simulink model "target_transmit"  (R2018a)
settings: Solver=FixedStepDiscrete  StartTime=0  StopTime=inf  RelTol=1e-3  EnableMultiTasking=on
InitFcn:
  | load data/bestsimulink_data
  | load data/bestsimulink320x240_data
  | load busObjects
StopFcn:
  | clear bestsimulink320x240_data
  | clear bestsimulink_data
  | clear dataBusObject
model workspace (MAT data in the model file):
  dt = 0.1
undefined symbols (not defined in the file or in its folder): gray, IsPositionTracked, IsSkeletonTracked, JointDepthIndices, JointImageIndices, JointTrackingState, JointWorldCoordinates, none, PositionDepthIndices, PositionImageIndices, PositionWorldCoordinates, Rec, SDTV, SegmentationData, SkeletonTrackingID, videoinput
libraries: visiontextngfix x24, embdlinuxlib x13, visionstatistics x7, visionconversions x5, visiontransforms x3, visionsinks x2, visionanalysis x1, dspvision x1, imaqlib x1, sldrtlib x1
(part 1 of 2)
settings Model: PauseTimes=118.9  ExtModeTrigDuration=100  Creator=sbiagion  LastModifiedBy=Farwa
settings DataIOCC: LimitDataPoints=on  SaveFormat=StructureWithTime
settings OptimizationCC: LifeSpan=1
settings DebuggingCC: UnderspecifiedInitializationDetection=Classic  MergeDetectMultiDrivingBlocksExec=none  SFUnexpectedBacktrackingDiag=warning  SFNoUnconditionalDefaultTransitionDiag=warning  SFExecutionAtInitializationDiag=none
settings HardwareCC: ProdBitPerPointer=32  ProdBitPerSizeT=32  ProdBitPerPtrDiffT=32  ProdLargestAtomicInteger=Long  ProdLargestAtomicFloat=Double  ProdIntDivRoundTo=Undefined  ProdWordSize=32  ProdHWDeviceType=ARM Compatible->ARM Cortex
settings ModelReferenceCC: PropagateSignalLabelsOutOfModel=off
settings SFSimCC: MATLABDynamicMemAlloc=off
settings RTWCC: SystemTargetFile=realtime.tlc  GenerateMakefile=off  TemplateMakefile=realtime.tmf  Description=Run on Target Hardware  RTWVerbose=off
settings CodeAppCC: StateflowObjectComments=on
settings STFCustomTargetCC: TargetLibSuffix=.a  GenerateSampleERTMain=on  ERTCustomFileBanners=on  SupportNonInlinedSFcns=off  RemoveResetFunc=on  SupportVariableSizeSignals=on  MATLABClassNameForMDSCustomization=Simulink.SoftwareTarget.ERTCustomization  GRTInterface=off  SystemTargetFile=realtime.tlc
settings ERTTargetCC: MultiwordLength=2048  GenerateSampleERTMain=on  ParMdlRefBuildCompliant=off  CompOptLevelCompliant=off  ConcurrentExecutionCompliant=off  CombineOutputUpdateFcns=off  SupportContinuousTime=on  SupportVariableSizeSignals=on  ModelStepFunctionPrototypeControlCompliant=off  CPPClassGenCompliant=off  UseToolchainInfoCompliant=off  ExtMode=on  ExtModeMexArgs='10.10.10.101' 0 17725  ERTSrcFileBannerTemplate=realtime_code_template.cgt  ERTHdrFileBannerTemplate=realtime_code_template.cgt  ERTDataSrcFileTemplate=realtime_code_template.cgt  ERTDataHdrFileTemplate=realtime_code_template.cgt  ERTCustomFileTemplate=realtime_file_process.tlc  ConvertIfToSwitch=off  SuppressUnreachableDefaultCases=off
settings ConfigComp: CovMetricSettings=dw  CovHtmlReporting=on  CovSaveCumulativeToWorkspaceVar=on  CovSaveSingleToWorkspaceVar=on  CovExternalEMLEnable=off

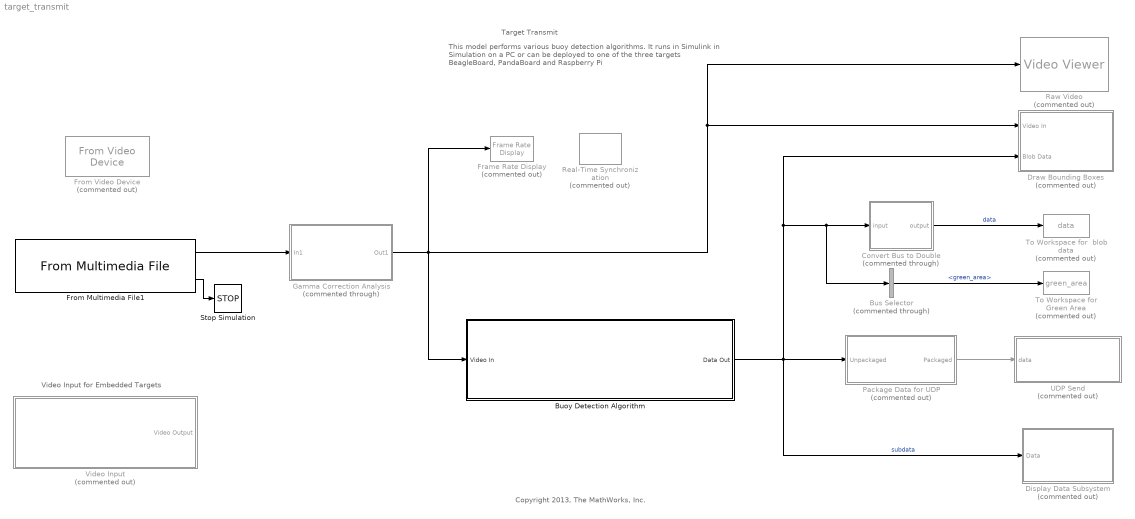
== system target_transmit ==
  note: This model performs various buoy detection algorithms.
      | It runs in Simulink in Simulation on a PC or can be deployed
      |  to one of the three targets BeagleBoard, PandaBoard and Raspberry Pi
  note: Target Transmit
  note: Copyright 2013, The MathWorks, Inc.
  note: Video Input for Embedded Targets
  Buoy Detection Algorithm : Subsystem  Variant=on  OverrideUsingVariant=testControl
  Bus Selector : BusSelector  Commented=through  OutputSignals=green_area
  Convert Bus to Double : Subsystem  Commented=through
  Display Data Subsystem : Subsystem  Commented=on
  Draw Bounding Boxes : Subsystem  Commented=on
  Frame Rate Display : visionsinks/Frame Rate Display  Commented=on  UpdateRate=10
      settings: SourceProductName=Computer Vision System Toolbox  SourceProductBaseCode=VP
  From Multimedia File1 : dspvision/From Multimedia File  inputFilename=E:\Actual_Computer_Stuff\Documents\RoboSoccer\soccer-vision\media\videos\2.mp4  loop=on  numPlays=1  outputStreams=Video only  videoDataType=single  audioDataType=int16  inheritSampleTime=on  userDefinedSampleTime=0.1  noAudioOutput=off  isIntensityVideo=off  fourcc=Intensity  colorVideoFormat=One multidimensional signal  outputEOF=on  dataOrg=Column-major  audioFrameSize=1024  computeAudioFrameSize=off  outSamplingMode=Sample based
      settings: SourceProductBaseCode=VP
  From Video Device : imaqlib/From Video Device  Commented=on  DeviceMenu=(none)  Device=winvideo 1 (Microsoft LifeCam Cinema)  ObjConstructor=videoinput('winvideo', 1)  VideoFormatMenu=(none)  VideoFormat=MJPG_640x480  VideoSource=input1  ROIPosition=[0 0 480 640]  EnableHWTrigger=off  TriggerConfiguration=none/none  SampleTime=0.1  OutputPortsMode=One multidimensional signal  DataType=single  CanDoHWTrigger=no  ReturnedColorSpace=rgb  BlockHandle=2792.0001  ROIWidth=640  ROIHeight=480  ROIColumn=0  ROIRow=0  EngXMLPath=C:\Program Files\MATLAB\R2018a\toolbox\imaq\imaq\private  DevXMLPath=C:\Program Files\MATLAB\R2015a\toolbox\imaq\imaqadaptors\win64  EngLibPath=C:\Program Files\MATLAB\R2018a\toolbox\imaq\imaqblks\imaqmex\win64  ColorSpace=rgb  BayerSensorAlignment=grbg  AllMetadata=IsPositionTracked;IsSkeletonTracked;JointDepthIndices;JointImageIndices;JointTrackingState;JointWorldCoordinates;PositionDepthIndices;PositionImageIndices;PositionWorldCoordinates;SegmentationData;SkeletonTrackingID
      settings: SourceProductName=Image Acquisition Toolbox
  Gamma Correction Analysis : Subsystem  Commented=through
  Package Data for UDP : Subsystem  Commented=on
  "Raw Video " : VideoViewer  Commented=on  colormapValue=gray(256)  FigPos=[1206 549 664 431]
  Real-Time Synchronization : sldrtlib/Real-Time Synchronization  Commented=on  SampleTime=0.1  MaxMissedTicks=1e9  ShowMissedTicks=off  YieldWhenWaiting=off
  Stop Simulation : Stop
  To Workspace for  blob data : ToWorkspace  Commented=on  VariableName=data  SaveFormat=Timeseries  SampleTime=-1
  To Workspace for Green Area : ToWorkspace  Commented=on  VariableName=green_area  SaveFormat=Structure With Time  SampleTime=-1
  UDP Send : Subsystem  Commented=on  Variant=on  OverrideUsingVariant=variantBeagle
  Video Input : Subsystem  Commented=on  Variant=on  OverrideUsingVariant=variantBeagle640x480
  wires:
  From Multimedia File1/2 -> Stop Simulation/1
  Buoy Detection Algorithm/1(Data Out) -> Draw Bounding Boxes/2(Blob Data), Bus Selector/1, Convert Bus to Double/1(input), Display Data Subsystem/1(Data), Package Data for UDP/1(Unpackaged)  "subdata"
  Convert Bus to Double/1(output) -> To Workspace for  blob data/1  "data"
  From Multimedia File1/1 -> Gamma Correction Analysis/1(In1)
  Gamma Correction Analysis/1(Out1) -> Frame Rate Display/1, "Raw Video "/1, Draw Bounding Boxes/1(Video In), Buoy Detection Algorithm/1(Video In)
  Package Data for UDP/1(Packaged) -> UDP Send/1(data)
  Bus Selector/1 -> To Workspace for Green Area/1  "<green_area>"

== system target_transmit/Buoy Detection Algorithm ==
  note: Lower and Upper Bound Thresholding for HSV
      | Multiple Threshold Sets
      | Simulink
      | - Thresholding
      | - Closing
      | - Blob Analysis
  note: Subtraction Based Thresholding in RGB
      | Simulink
      | - Thresholding
      | - Blob Analysis
      | - Limited to 4 Blobs
  note: Lower and Upper Bound Thresholding for RGB
      | Multiple Threshold Sets
      | Matlab Function Block
      | - Thresholding
      | - Closing
      | - Blob Analysis
  note: Lower and Upper Bound Based Thresholding for RGB
      | Multiple Threshold Sets
      | Matlab Function Block
      | - Thresholding
      | - Blob Analysis
  note: Lower and Upper Bound Based Thresholding for RGB
      | Multiple Threshold Sets
      | Simulink
      | - Thresholding
      | - Blob Analysis
  note: Lower and Upper Bound Based Thresholding for RGB
      | Single Threshold Set
      | Simulink
      | - Thresholding
      | - Blob Analysis
  note: Lower and Upper Bound Thresholding for RGB
      | Multiple Threshold Sets
      | Simulink
      | - Thresholding
      | - Closing
      | - Blob Analysis
  note: Subtraction Based Thresholding in RGB
      | Simulink
      | - Thresholding
      | - Blob Analysis
      | - Limited to 50 Blobs
  Video In : Inport
  variant1: Subtraction Based Thresholding 4 Blobs : Subsystem  VariantControl=testControl
  Data Out : Outport

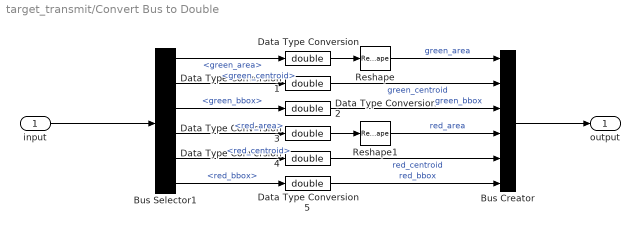
== system target_transmit/Convert Bus to Double ==
  input : Inport
  Bus Creator : BusCreator  Inputs=6
  Bus Selector1 : BusSelector  OutputSignals=green_area,green_centroid,green_bbox,red_area,red_centroid,red_bbox
  Data Type Conversion{,1..5} (6 alike) : DataTypeConversion  OutDataTypeStr=double
  Reshape : Reshape
  Reshape1 : Reshape
  output : Outport
  wires:
  Bus Creator/1 -> output/1
  input/1 -> Bus Selector1/1
  Bus Selector1/4 -> Data Type Conversion3/1  "<red_area>"
  Bus Selector1/6 -> Data Type Conversion5/1  "<red_bbox>"
  Bus Selector1/5 -> Data Type Conversion4/1  "<red_centroid>"
  Bus Selector1/2 -> Data Type Conversion1/1  "<green_centroid>"
  Bus Selector1/3 -> Data Type Conversion2/1  "<green_bbox>"
  Bus Selector1/1 -> Data Type Conversion/1  "<green_area>"
  Data Type Conversion/1 -> Reshape/1
  Data Type Conversion1/1 -> Bus Creator/2  "green_centroid"
  Data Type Conversion2/1 -> Bus Creator/3  "green_bbox"
  Data Type Conversion3/1 -> Reshape1/1
  Data Type Conversion4/1 -> Bus Creator/5  "red_centroid"
  Data Type Conversion5/1 -> Bus Creator/6  "red_bbox"
  Reshape/1 -> Bus Creator/1  "green_area"
  Reshape1/1 -> Bus Creator/4  "red_area"

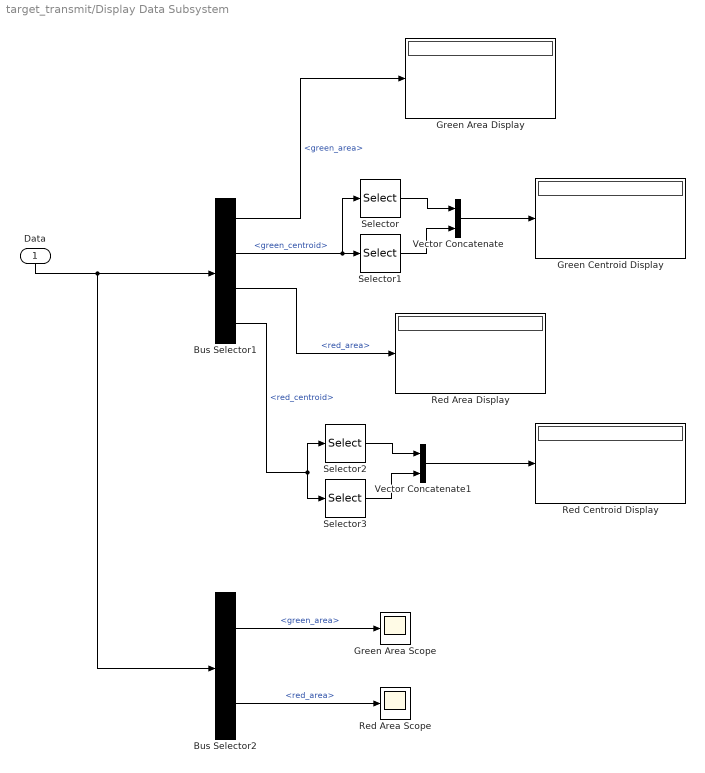
== system target_transmit/Display Data Subsystem ==
  Data : Inport
  Bus Selector1 : BusSelector  OutputSignals=green_area,green_centroid,red_area,red_centroid
  Bus Selector2 : BusSelector  OutputSignals=green_area,red_area
  Green Area Display : Display
  Green Area Scope : Scope
  Green Centroid Display : Display
  Red Area Display : Display
  Red Area Scope : Scope
  Red Centroid Display : Display
  Selector : Selector  NumberOfDimensions=2  InputPortWidth=3  IndexOptions=Select all,Index vector (dialog)  Indices=[1 3],2  OutputSizes=1,1
  Selector1 : Selector  NumberOfDimensions=2  InputPortWidth=3  IndexOptions=Select all,Index vector (dialog)  Indices=[1 3],1  OutputSizes=1,1
  Selector2 : Selector  NumberOfDimensions=2  InputPortWidth=3  IndexOptions=Select all,Index vector (dialog)  Indices=[1 3],2  OutputSizes=1,1
  Selector3 : Selector  NumberOfDimensions=2  InputPortWidth=3  IndexOptions=Select all,Index vector (dialog)  Indices=[1 3],1  OutputSizes=1,1
  Vector Concatenate : Concatenate  Mode=Multidimensional array  ConcatenateDimension=2
  Vector Concatenate1 : Concatenate  Mode=Multidimensional array  ConcatenateDimension=2
  wires:
  Data/1 -> Bus Selector2/1, Bus Selector1/1
  Bus Selector1/1 -> Green Area Display/1  "<green_area>"
  Bus Selector1/2 -> Selector1/1, Selector/1  "<green_centroid>"
  Bus Selector1/3 -> Red Area Display/1  "<red_area>"
  Bus Selector2/1 -> Green Area Scope/1  "<green_area>"
  Bus Selector2/2 -> Red Area Scope/1  "<red_area>"
  Selector/1 -> Vector Concatenate/1
  Selector1/1 -> Vector Concatenate/2
  Vector Concatenate/1 -> Green Centroid Display/1
  Bus Selector1/4 -> Selector3/1, Selector2/1  "<red_centroid>"
  Selector2/1 -> Vector Concatenate1/1
  Selector3/1 -> Vector Concatenate1/2
  Vector Concatenate1/1 -> Red Centroid Display/1

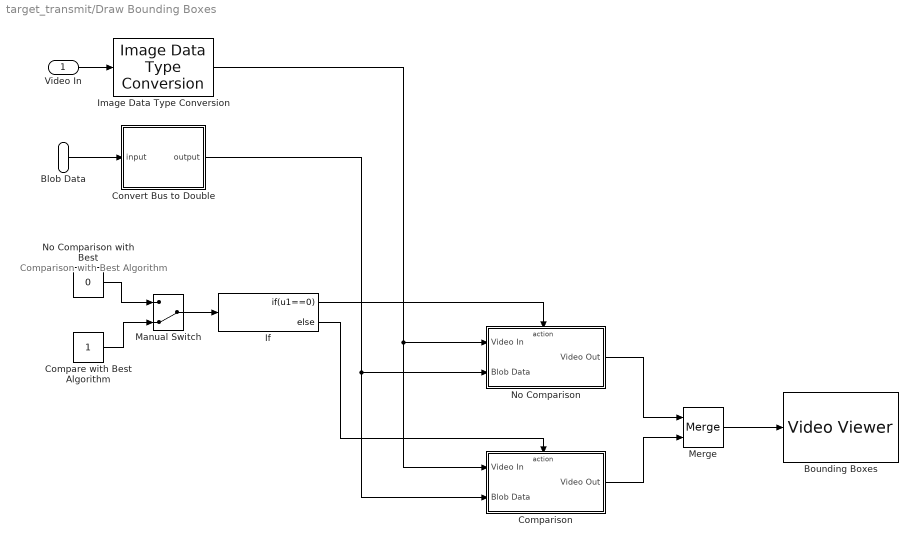
== system target_transmit/Draw Bounding Boxes ==
  note: Comparison with Best Algorithm
  Video In : Inport
  Blob Data : Inport  Port=2
  Bounding Boxes : VideoViewer  colormapValue=gray(256)  FigPos=[1 678 1280 582.666666666667]
  Compare with Best Algorithm : Constant
  Comparison : Subsystem  TreatAsAtomicUnit=on
  Convert Bus to Double : Subsystem
  If : If  IfExpression=u1==0
  Image Data Type Conversion : visionconversions/Image Data Type Conversion  outDT=double  isSigned=on  wordLen=16  numFracBits=0
      settings: SourceProductName=Computer Vision System Toolbox  SourceProductBaseCode=VP
  Manual Switch : ManualSwitch  CurrentSetting=0
  Merge : Merge
  No Comparison : Subsystem  TreatAsAtomicUnit=on
  No Comparison with Best : Constant  Value=0
  wires:
  Video In/1 -> Image Data Type Conversion/1
  Blob Data/1 -> Convert Bus to Double/1(input)
  Convert Bus to Double/1(output) -> No Comparison/2(Blob Data), Comparison/2(Blob Data)
  No Comparison with Best/1 -> Manual Switch/1
  Compare with Best Algorithm/1 -> Manual Switch/2
  Manual Switch/1 -> If/1
  If/1 -> No Comparison/Action
  Image Data Type Conversion/1 -> Comparison/1(Video In), No Comparison/1(Video In)
  If/2 -> Comparison/Action
  No Comparison/1(Video Out) -> Merge/1
  Comparison/1(Video Out) -> Merge/2
  Merge/1 -> Bounding Boxes/1

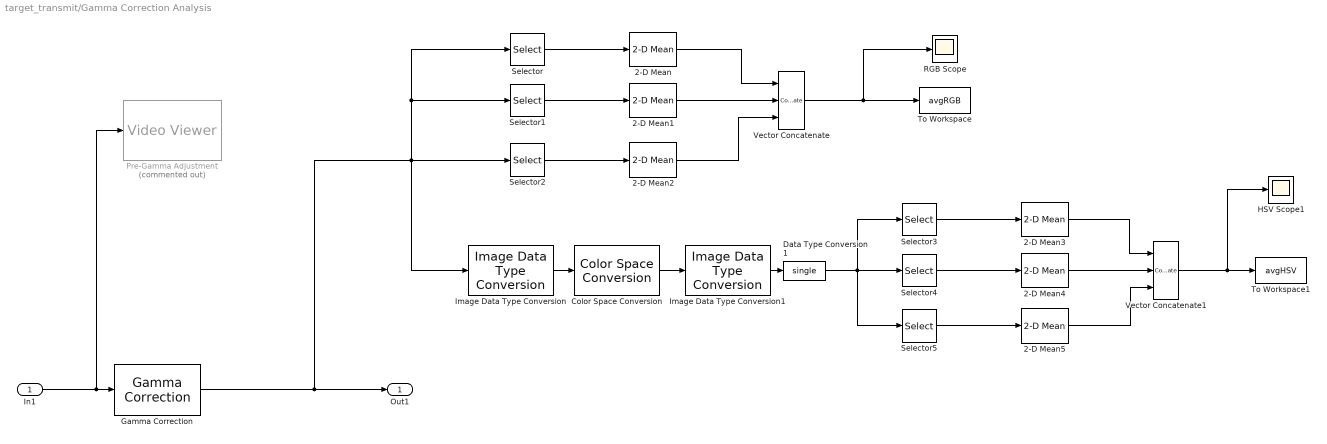
== system target_transmit/Gamma Correction Analysis ==
  In1 : Inport
  2-D Mean{,1..5} (6 alike) : visionstatistics/2-D Mean  run=off  reset_popup=None  directionMode=Entire input  dimension=1  treatSBRowAsCol=on  roiEnable=off  roiType=Rectangles  roiPortion=Entire ROI  roiOutput=Individual statistics for each ROI  roiFlag=off  outputDataTypeStr=Inherit: Same as accumulator  outputLastDataTypeStr=Inherit: Same as accumulator  outputMin=[]  outputMax=[]  accumMode=Binary point scaling  accumWordLength=32  accumFracLength=0  accumDataTypeStr=fixdt([],32,0)  accumLastDataTypeStr=fixdt([],32,0)  roundingMode=Floor  overflowMode=off
      settings: SourceProductName=Computer Vision System Toolbox  SourceProductBaseCode=VP
  Color Space Conversion : visionconversions/Color Space  Conversion  conversion=Obsolete  conversionActive=R'G'B' to HSV  wp_str=D65  rec=Rec. 601 (SDTV)  sys=1125/60/2:1  imagePorts=One multidimensional signal
      settings: SourceProductName=Computer Vision System Toolbox
  Data Type Conversion1 : DataTypeConversion  OutDataTypeStr=single  SaturateOnIntegerOverflow=on  RndMeth=Zero
  Gamma Correction : visionconversions/Gamma Correction  operation=Gamma  gamma=1.5  linearSegment=on  breakPoint=0.018
      settings: SourceProductName=Computer Vision System Toolbox  SourceProductBaseCode=VP
  HSV Scope1 : Scope
  Image Data Type Conversion : visionconversions/Image Data Type Conversion  outDT=single  isSigned=on  wordLen=16  numFracBits=0
      settings: SourceProductName=Computer Vision System Toolbox  SourceProductBaseCode=VP
  Image Data Type Conversion1 : visionconversions/Image Data Type Conversion  outDT=uint8  isSigned=on  wordLen=16  numFracBits=0
      settings: SourceProductName=Computer Vision System Toolbox  SourceProductBaseCode=VP
  Pre-Gamma Adjustment : visionsinks/Video Viewer  Commented=on  inputType=Obsolete7b  imagePorts=One multidimensional signal  useColorMap=off  colormapValue=gray(256)  specRange=off  minInputVal=0  maxInputVal=255  FigPos=[119 991 1008 708]  AxisZoom=on  trueSizedOnce=off  OpenAtMdlStart=on  DefaultConfigurationName=vipscopes.VideoViewerScopeCfg
      settings: SourceProductName=Computer Vision System Toolbox  SourceProductBaseCode=VP
  RGB Scope : Scope
  Selector : Selector  NumberOfDimensions=3  InputPortWidth=3  IndexOptions=Select all,Select all,Index vector (dialog)  Indices=[1 3],1,1  OutputSizes=1,1,1
  Selector1 : Selector  NumberOfDimensions=3  InputPortWidth=3  IndexOptions=Select all,Select all,Index vector (dialog)  Indices=[1 3],1,2  OutputSizes=1,1,1
  Selector2 : Selector  NumberOfDimensions=3  InputPortWidth=3  IndexOptions=Select all,Select all,Index vector (dialog)  Indices=[1 3],1,3  OutputSizes=1,1,1
  Selector3 : Selector  NumberOfDimensions=3  InputPortWidth=3  IndexOptions=Select all,Select all,Index vector (dialog)  Indices=[1 3],1,1  OutputSizes=1,1,1
  Selector4 : Selector  NumberOfDimensions=3  InputPortWidth=3  IndexOptions=Select all,Select all,Index vector (dialog)  Indices=[1 3],1,2  OutputSizes=1,1,1
  Selector5 : Selector  NumberOfDimensions=3  InputPortWidth=3  IndexOptions=Select all,Select all,Index vector (dialog)  Indices=[1 3],1,3  OutputSizes=1,1,1
  To Workspace : ToWorkspace  VariableName=avgRGB  SaveFormat=Timeseries  SampleTime=-1
  To Workspace1 : ToWorkspace  VariableName=avgHSV  SaveFormat=Timeseries  SampleTime=-1
  Vector Concatenate : Concatenate  NumInputs=3
  Vector Concatenate1 : Concatenate  NumInputs=3
  Out1 : Outport
  wires:
  In1/1 -> Pre-Gamma Adjustment/1, Gamma Correction/1
  Gamma Correction/1 -> Selector2/1, Selector1/1, Selector/1, Image Data Type Conversion/1, Out1/1
  Selector1/1 -> 2-D Mean1/1
  Selector2/1 -> 2-D Mean2/1
  Selector/1 -> 2-D Mean/1
  2-D Mean/1 -> Vector Concatenate/1
  2-D Mean1/1 -> Vector Concatenate/2
  2-D Mean2/1 -> Vector Concatenate/3
  Vector Concatenate/1 -> To Workspace/1, RGB Scope/1
  Color Space Conversion/1 -> Image Data Type Conversion1/1
  Image Data Type Conversion/1 -> Color Space Conversion/1
  Data Type Conversion1/1 -> Selector5/1, Selector3/1, Selector4/1
  2-D Mean3/1 -> Vector Concatenate1/1
  2-D Mean4/1 -> Vector Concatenate1/2
  2-D Mean5/1 -> Vector Concatenate1/3
  Vector Concatenate1/1 -> HSV Scope1/1, To Workspace1/1
  Selector3/1 -> 2-D Mean3/1
  Selector4/1 -> 2-D Mean4/1
  Selector5/1 -> 2-D Mean5/1
  Image Data Type Conversion1/1 -> Data Type Conversion1/1

== system target_transmit/Package Data for UDP ==
  Unpackaged : Inport
  Bus Selector : BusSelector  OutputSignals=green_area,green_centroid,red_area,red_centroid
  Mux : Mux
  Reshape1 : Reshape
  Reshape2 : Reshape
  Packaged : Outport
  wires:
  Mux/1 -> Packaged/1
  Bus Selector/1 -> Mux/1  "<green_area>"
  Bus Selector/2 -> Reshape2/1  "<green_centroid>"
  Bus Selector/3 -> Mux/3  "<red_area>"
  Bus Selector/4 -> Reshape1/1  "<red_centroid>"
  Reshape2/1 -> Mux/2
  Reshape1/1 -> Mux/4
  Unpackaged/1 -> Bus Selector/1

== system target_transmit/UDP Send ==
  data : Inport
  UDP Send BeagleBoard : Subsystem  VariantControl=variantBeagle
  UDP Send PandaBoard : Subsystem  VariantControl=variantPanda
  UDP Send RaspberryPi : Subsystem  VariantControl=variantRPi

== system target_transmit/Video Input ==
  variant1: BeagleBoard 640x480 : Subsystem  VariantControl=variantBeagle640x480
  variant2: BeagleBoard 320x240 : Subsystem  VariantControl=variantBeagle320x240
  variant3: PandaBoard 640x480 : Subsystem  VariantControl=variantPanda640x480
  variant4: PandaBoard 320x240 : Subsystem  VariantControl=variantPanda320x240
  variant5: RasbPi 320x240 : Subsystem  VariantControl=variantRasbPi320x240
  Video Output : Outport

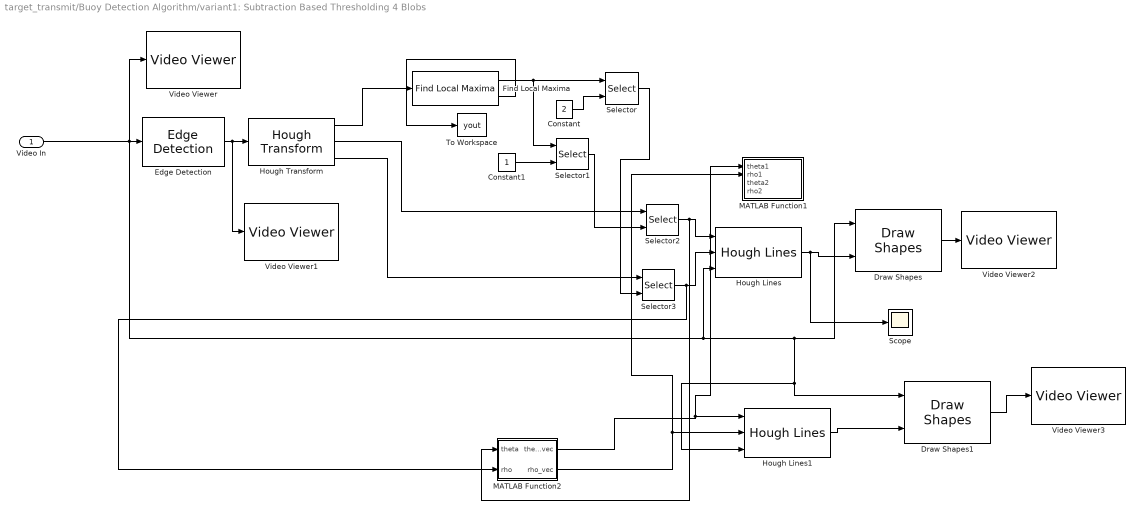
== system target_transmit/Buoy Detection Algorithm/variant1: Subtraction Based Thresholding 4 Blobs ==
  Video In : Inport
  Constant : Constant  Value=2
  Constant1 : Constant
  Draw Shapes : visiontextngfix/Draw Shapes  shape=Lines  fill=off  lineWidth=8  fillClrSource=Specify via dialog  display=White  intensity=200  color=[0 128 0]  opacity=0.6  viewport=Entire image  antialiasing=off  inType=Obsolete  imagePorts=One multidimensional signal  prodOutputMode=Binary point scaling  prodOutputWordLength=32  prodOutputFracLength=14  memoryMode=Specify word length  memoryWordLength=16  memoryFracLength=14  roundingMode=Floor  overflowMode=off
      settings: SourceProductName=Computer Vision System Toolbox
  Draw Shapes1 : visiontextngfix/Draw Shapes  shape=Lines  fill=off  lineWidth=8  fillClrSource=Specify via dialog  display=Black  intensity=200  color=[0 128 0]  opacity=0.6  viewport=Entire image  antialiasing=off  inType=Obsolete  imagePorts=One multidimensional signal  prodOutputMode=Binary point scaling  prodOutputWordLength=32  prodOutputFracLength=14  memoryMode=Specify word length  memoryWordLength=16  memoryFracLength=14  roundingMode=Floor  overflowMode=off
      settings: SourceProductName=Computer Vision System Toolbox
  Edge Detection : visionanalysis/Edge Detection  method=Sobel  outputType=Binary image  userDefinedThreshold=off  thresholdSource=Input port  threshold=20  thresholdTuning=12  edgeThinning=off  threshold_canny=[0.25 0.60]  autoPercent=70  sigma=1  roundingMode=Floor  overflowMode=off  prodOutputMode=Binary point scaling  prodOutputWordLength=32  prodOutputFracLength=8  prodOutputSlope=2^-8  accumSlope=2^-8  outputSlope=2^-4
      settings: SourceProductName=Computer Vision System Toolbox  SourceProductBaseCode=VP
  Find Local Maxima : visionstatistics/Find Local Maxima  num_peaks=8  nhood_size=[5 7]  src_thresh=Obsolete9b  src_thresh_inuse=Specify via dialog  threshold=10  inputIsHough=on  dt_peak=uint32  isOutVarDim=off  dt_count=uint32
      settings: SourceProductName=Computer Vision System Toolbox  SourceProductBaseCode=VP
  Hough Lines : visiontransforms/Hough Lines  sineCompMethod=Trigonometric function  thetaRes=pi/180  firstCoeffMode=Specify word length  firstCoeffWordLength=16  firstCoeffFracLength=15  prodOutputMode=Binary point scaling  prodOutputWordLength=32  prodOutputFracLength=16  roundingMode=Nearest  overflowMode=on
      settings: SourceProductName=Computer Vision System Toolbox  SourceProductBaseCode=VP
  Hough Lines1 : visiontransforms/Hough Lines  sineCompMethod=Trigonometric function  thetaRes=pi/180  firstCoeffMode=Specify word length  firstCoeffWordLength=16  firstCoeffFracLength=15  prodOutputMode=Binary point scaling  prodOutputWordLength=32  prodOutputFracLength=16  roundingMode=Nearest  overflowMode=on
      settings: SourceProductName=Computer Vision System Toolbox  SourceProductBaseCode=VP
  Hough Transform : visiontransforms/Hough Transform  theta_res=pi/360  rho_res=1  out_theta_rho=on  outdtmode=double  firstCoeffMode=Binary point scaling  firstCoeffWordLength=16  firstCoeffFracLength=14  secondCoeffMode=Binary point scaling  secondCoeffWordLength=32  secondCoeffFracLength=16  outputMode=Binary point scaling  outputWordLength=16  outputFracLength=0  accumMode=Binary point scaling  accumWordLength=32  accumFracLength=20  prodOutputMode=Binary point scaling  prodOutputWordLength=32  prodOutputFracLength=20  memoryMode=Binary point scaling  memoryWordLength=32  memoryFracLength=16  roundingMode=Nearest  overflowMode=on
      settings: SourceProductName=Computer Vision System Toolbox  SourceProductBaseCode=VP
  MATLAB Function1 : MATLAB Function  TreatAsAtomicUnit=on
  MATLAB Function2 : MATLAB Function  TreatAsAtomicUnit=on
  Scope : Scope
  Selector : Selector  NumberOfDimensions=2  InputPortWidth=2  IndexOptions=Select all,Index vector (port)  Indices=1,1  OutputSizes=1,1
  Selector1 : Selector  NumberOfDimensions=2  InputPortWidth=2  IndexOptions=Select all,Index vector (port)  Indices=0,1  OutputSizes=1,1
  Selector2 : Selector  NumberOfDimensions=2  InputPortWidth=3  IndexOptions=Select all,Index vector (port)  Indices=[1 3],1  OutputSizes=1,1
  Selector3 : Selector  NumberOfDimensions=2  InputPortWidth=3  IndexOptions=Select all,Index vector (port)  Indices=[1 3],1  OutputSizes=1,1
  To Workspace : ToWorkspace  VariableName=yout  SampleTime=-1
      settings: Save2DSignal=2-D array (concatenate along first dimension)
  Video Viewer : VideoViewer  colormapValue=gray(256)  FigPos=[1 678 1280 582.666666666667]
  Video Viewer1 : VideoViewer  colormapValue=gray(256)  FigPos=[1 678 1280 582.666666666667]
  Video Viewer2 : VideoViewer  colormapValue=gray(256)  FigPos=[503.666666666667 715.333333333333 638.666666666667 574.666666666667]
  Video Viewer3 : VideoViewer  colormapValue=gray(256)  FigPos=[-11.6666666666667 725.333333333333 1280 582.666666666667]
  wires:
  Constant1/1 -> Selector1/2
  Video In/1 -> Edge Detection/1, Hough Lines/3, Draw Shapes1/1, Hough Lines1/3, Draw Shapes/1, Video Viewer/1
  Hough Lines/1 -> Scope/1, Draw Shapes/2
  Selector/1 -> Selector3/2
  Selector1/1 -> Selector2/2
  Draw Shapes/1 -> Video Viewer2/1
  Find Local Maxima/1 -> Selector1/1, Selector/1
  Hough Transform/2 -> Selector2/1
  Constant/1 -> Selector/2
  Edge Detection/1 -> Hough Transform/1, Video Viewer1/1
  Hough Transform/1 -> Find Local Maxima/1
  Find Local Maxima/2 -> To Workspace/1
  Selector3/1 -> MATLAB Function2/2(rho), Hough Lines/2
  Selector2/1 -> MATLAB Function2/1(theta), Hough Lines/1
  Hough Transform/3 -> Selector3/1
  Draw Shapes1/1 -> Video Viewer3/1
  Hough Lines1/1 -> Draw Shapes1/2
  MATLAB Function2/1(theta_vec) -> MATLAB Function1/1(theta1), Hough Lines1/1
  MATLAB Function2/2(rho_vec) -> MATLAB Function1/2(rho1), Hough Lines1/2

== system target_transmit/Draw Bounding Boxes/Comparison ==
  Video In : Inport
  Blob Data : Inport  Port=2
  Action Port : ActionPort  ActionType=else
  Insert Algorithm Blobs : Subsystem
  Insert Area Text : Subsystem  Commented=through
  Insert Best Algorithm Blobs : Subsystem
  Insert Closest Text : Subsystem
  Insert Speed Gate or Buoy Text : Subsystem  Commented=through
  Reflection Removal : Subsystem  Commented=through
  Video Out : Outport
  wires:
  Blob Data/1 -> Reflection Removal/1(Blob Data In)
  Video In/1 -> Insert Best Algorithm Blobs/1(Video In)
  Insert Best Algorithm Blobs/1(Video Out) -> Insert Closest Text/1(Video In)
  Reflection Removal/1(Blob Data Out) -> Insert Area Text/2(Blob Data)
  Insert Closest Text/1(Video Out) -> Insert Area Text/1(Video In)
  Insert Area Text/1(Video Out) -> Insert Speed Gate or Buoy Text/1(Video In)
  Insert Speed Gate or Buoy Text/1(Video Out) -> Insert Algorithm Blobs/1(Video In)
  Insert Algorithm Blobs/1(Video Out) -> Video Out/1
  Insert Speed Gate or Buoy Text/2(Data output) -> Insert Algorithm Blobs/2(Blob Data)
  Insert Area Text/2(Blob Data Out) -> Insert Speed Gate or Buoy Text/2(Blob Data)
  Insert Best Algorithm Blobs/2(Best Data Out) -> Insert Closest Text/2(Blob Data)

== system target_transmit/Draw Bounding Boxes/Convert Bus to Double ==
  input : Inport
  Bus Creator : BusCreator  Inputs=6
  Bus Selector1 : BusSelector  OutputSignals=green_area,green_centroid,green_bbox,red_area,red_centroid,red_bbox
  Data Type Conversion{,1..5} (6 alike) : DataTypeConversion  OutDataTypeStr=double
  output : Outport
  wires:
  Bus Creator/1 -> output/1
  input/1 -> Bus Selector1/1
  Bus Selector1/4 -> Data Type Conversion3/1  "<red_area>"
  Bus Selector1/6 -> Data Type Conversion5/1  "<red_bbox>"
  Bus Selector1/5 -> Data Type Conversion4/1  "<red_centroid>"
  Bus Selector1/2 -> Data Type Conversion1/1  "<green_centroid>"
  Bus Selector1/3 -> Data Type Conversion2/1  "<green_bbox>"
  Bus Selector1/1 -> Data Type Conversion/1  "<green_area>"
  Data Type Conversion1/1 -> Bus Creator/2  "green_centroid"
  Data Type Conversion2/1 -> Bus Creator/3  "green_bbox"
  Data Type Conversion4/1 -> Bus Creator/5  "red_centroid"
  Data Type Conversion5/1 -> Bus Creator/6  "red_bbox"
  Data Type Conversion/1 -> Bus Creator/1  "green_area"
  Data Type Conversion3/1 -> Bus Creator/4  "red_area"

== system target_transmit/Draw Bounding Boxes/No Comparison ==
  Video In : Inport
  Blob Data : Inport  Port=2
  Action Port : ActionPort  ActionType=then
  Insert Area Text : Subsystem  Commented=through
  Insert Buoy Blobs1 : Subsystem
  Insert Closest Text : Subsystem
  Insert Speed Gate or Buoy Text : Subsystem  Commented=through
  Reflection Removal : Subsystem  Commented=through
  Video Out : Outport
  wires:
  Insert Area Text/1(Video Out) -> Insert Speed Gate or Buoy Text/1(Video In)
  Insert Closest Text/1(Video Out) -> Insert Area Text/1(Video In)
  Insert Speed Gate or Buoy Text/1(Video Out) -> Video Out/1
  Reflection Removal/1(Blob Data Out) -> Insert Buoy Blobs1/2(Blob Data), Insert Area Text/2(Blob Data), Insert Closest Text/2(Blob Data)
  Insert Buoy Blobs1/1(Video Out) -> Insert Closest Text/1(Video In)
  Video In/1 -> Insert Buoy Blobs1/1(Video In)
  Blob Data/1 -> Reflection Removal/1(Blob Data In)
  Insert Area Text/2(Blob Data Out) -> Insert Speed Gate or Buoy Text/2(Blob Data)

== system target_transmit/UDP Send/UDP Send BeagleBoard ==
  data : Inport
  UDP Send : embdlinuxlib/UDP Send  remoteURL='10.10.10.100'  remotePort=25001  localURL='255.255.255.255'  localPortSource=Automatically determine  localPort=-1  sampletime=-1  blockPlatform=BeagleBoard  separateLengthPort=0
      settings: SourceProductName=Simulink Support Package for Raspberry Pi Hardware  SourceProductBaseCode=RASPPI
  wires:
  data/1 -> UDP Send/1

== system target_transmit/UDP Send/UDP Send PandaBoard ==
  data : Inport
  UDP Send1 : embdlinuxlib/UDP Send  remoteURL='10.10.10.100'  remotePort=25001  localURL='255.255.255.255'  localPortSource=Automatically determine  localPort=-1  sampletime=-1  blockPlatform=PandaBoard  separateLengthPort=0
      settings: SourceProductName=Simulink Support Package for Raspberry Pi Hardware  SourceProductBaseCode=RASPPI
  wires:
  data/1 -> UDP Send1/1

== system target_transmit/UDP Send/UDP Send RaspberryPi ==
  data : Inport
  UDP Send2 : embdlinuxlib/UDP Send  remoteURL='172.28.65.74'  remotePort=25000  localURL='255.255.255.255'  localPortSource=Automatically determine  localPort=-1  sampletime=-1  blockPlatform=Raspberry Pi  separateLengthPort=0
      settings: SourceProductName=Simulink Support Package for Raspberry Pi Hardware  SourceProductBaseCode=RASPPI
  wires:
  data/1 -> UDP Send2/1

== system target_transmit/Video Input/variant1: BeagleBoard 640x480 ==
  SDL Video Display : embdlinuxlib/SDL Video Display  Commented=on  pixelFormat=RGB  pixelOrder=Planar  rowMajor=on  blockPlatform=BeagleBoard
      settings: SourceProductName=Simulink Support Package for Raspberry Pi Hardware  SourceProductBaseCode=RASPPI
  V4L2 Video Capture : embdlinuxlib/V4L2 Video Capture  m_devName='/dev/video0'  roi=[0, 0, 640, 480]  imSizeSelection=640x480  imSize=[640, 480]  pixelFormat=RGB  pixelOrder=Planar  sampleTime=0.1  simOutput=Colorbars  blockPlatform=BeagleBoard
      settings: SourceProductName=Simulink Support Package for Raspberry Pi Hardware  SourceProductBaseCode=RASPPI
  Vector Concatenate : Concatenate  NumInputs=3  Mode=Multidimensional array  ConcatenateDimension=3
  Video Output : Outport
  wires:
  Vector Concatenate/1 -> Video Output/1
  V4L2 Video Capture/1 -> SDL Video Display/1, Vector Concatenate/1
  V4L2 Video Capture/2 -> SDL Video Display/2, Vector Concatenate/2
  V4L2 Video Capture/3 -> SDL Video Display/3, Vector Concatenate/3

== system target_transmit/Video Input/variant2: BeagleBoard 320x240 ==
  SDL Video Display : embdlinuxlib/SDL Video Display  pixelFormat=RGB  pixelOrder=Planar  rowMajor=on  blockPlatform=BeagleBoard
      settings: SourceProductName=Simulink Support Package for Raspberry Pi Hardware  SourceProductBaseCode=RASPPI
  V4L2 Video Capture : embdlinuxlib/V4L2 Video Capture  m_devName='/dev/video0'  roi=[0, 0, 640, 480]  imSizeSelection=320x240  imSize=[640, 480]  pixelFormat=RGB  pixelOrder=Planar  sampleTime=0.1  simOutput=Colorbars  blockPlatform=BeagleBoard
      settings: SourceProductName=Simulink Support Package for Raspberry Pi Hardware  SourceProductBaseCode=RASPPI
  Vector Concatenate : Concatenate  NumInputs=3  Mode=Multidimensional array  ConcatenateDimension=3
  Video Output : Outport
  wires:
  V4L2 Video Capture/3 -> Vector Concatenate/3, SDL Video Display/3
  V4L2 Video Capture/2 -> Vector Concatenate/2, SDL Video Display/2
  V4L2 Video Capture/1 -> Vector Concatenate/1, SDL Video Display/1
  Vector Concatenate/1 -> Video Output/1

== system target_transmit/Video Input/variant3: PandaBoard 640x480 ==
  SDL Video Display : embdlinuxlib/SDL Video Display  pixelFormat=RGB  pixelOrder=Planar  rowMajor=on  blockPlatform=PandaBoard
      settings: SourceProductName=Simulink Support Package for Raspberry Pi Hardware  SourceProductBaseCode=RASPPI
  V4L2 Video Capture1 : embdlinuxlib/V4L2 Video Capture  m_devName='/dev/video3'  roi=[0, 0, 640, 480]  imSizeSelection=640x480  imSize=[640, 480]  pixelFormat=RGB  pixelOrder=Planar  sampleTime=0.1  simOutput=Colorbars  blockPlatform=PandaBoard
      settings: SourceProductName=Simulink Support Package for Raspberry Pi Hardware  SourceProductBaseCode=RASPPI
  Vector Concatenate1 : Concatenate  NumInputs=3  Mode=Multidimensional array  ConcatenateDimension=3
  Video Output : Outport
  wires:
  Vector Concatenate1/1 -> Video Output/1
  V4L2 Video Capture1/3 -> SDL Video Display/3, Vector Concatenate1/3
  V4L2 Video Capture1/1 -> SDL Video Display/1, Vector Concatenate1/1
  V4L2 Video Capture1/2 -> SDL Video Display/2, Vector Concatenate1/2

== system target_transmit/Video Input/variant4: PandaBoard 320x240 ==
  SDL Video Display : embdlinuxlib/SDL Video Display  pixelFormat=RGB  pixelOrder=Planar  rowMajor=on  blockPlatform=PandaBoard
      settings: SourceProductName=Simulink Support Package for Raspberry Pi Hardware  SourceProductBaseCode=RASPPI
  V4L2 Video Capture1 : embdlinuxlib/V4L2 Video Capture  m_devName='/dev/video3'  roi=[0, 0, 640, 480]  imSizeSelection=320x240  imSize=[640, 480]  pixelFormat=RGB  pixelOrder=Planar  sampleTime=0.5  simOutput=Colorbars  blockPlatform=PandaBoard
      settings: SourceProductName=Simulink Support Package for Raspberry Pi Hardware  SourceProductBaseCode=RASPPI
  Vector Concatenate1 : Concatenate  NumInputs=3  Mode=Multidimensional array  ConcatenateDimension=3
  Video Output : Outport
  wires:
  V4L2 Video Capture1/2 -> Vector Concatenate1/2, SDL Video Display/2
  V4L2 Video Capture1/1 -> Vector Concatenate1/1, SDL Video Display/1
  V4L2 Video Capture1/3 -> Vector Concatenate1/3, SDL Video Display/3
  Vector Concatenate1/1 -> Video Output/1

== system target_transmit/Video Input/variant5: RasbPi 320x240 ==
  SDL Video Display1 : embdlinuxlib/SDL Video Display  pixelFormat=RGB  pixelOrder=Planar  rowMajor=on  blockPlatform=Raspberry Pi
      settings: SourceProductName=Simulink Support Package for Raspberry Pi Hardware  SourceProductBaseCode=RASPPI
  V4L2 Video Capture2 : embdlinuxlib/V4L2 Video Capture  m_devName='/dev/video0'  roi=[0, 0, 640, 480]  imSizeSelection=320x240  imSize=[640, 480]  pixelFormat=RGB  pixelOrder=Planar  sampleTime=0.1  simOutput=Colorbars  blockPlatform=Raspberry Pi
      settings: SourceProductName=Simulink Support Package for Raspberry Pi Hardware  SourceProductBaseCode=RASPPI
  Vector Concatenate2 : Concatenate  NumInputs=3  Mode=Multidimensional array  ConcatenateDimension=3
  Video Output : Outport
  wires:
  V4L2 Video Capture2/1 -> Vector Concatenate2/1, SDL Video Display1/1
  V4L2 Video Capture2/2 -> Vector Concatenate2/2, SDL Video Display1/2
  V4L2 Video Capture2/3 -> Vector Concatenate2/3, SDL Video Display1/3
  Vector Concatenate2/1 -> Video Output/1

== system target_transmit/Draw Bounding Boxes/Comparison/Insert Algorithm Blobs ==
  Video In : Inport
  Blob Data : Inport  Port=2
  Bus Selector : BusSelector  OutputSignals=green_bbox,red_bbox
  Draw Shapes Green : visiontextngfix/Draw Shapes  shape=Rectangles  fill=off  lineWidth=1  fillClrSource=Specify via dialog  display=Black  intensity=200  color=[0 255 0]  opacity=0.6  viewport=Entire image  antialiasing=off  inType=Obsolete  imagePorts=One multidimensional signal  prodOutputMode=Binary point scaling  prodOutputWordLength=32  prodOutputFracLength=14  memoryMode=Specify word length  memoryWordLength=16  memoryFracLength=14  roundingMode=Floor  overflowMode=off
      settings: SourceProductName=Computer Vision System Toolbox
  Draw Shapes Red : visiontextngfix/Draw Shapes  shape=Rectangles  fill=off  lineWidth=1  fillClrSource=Specify via dialog  display=Black  intensity=200  color=[255 0 0]  opacity=0.6  viewport=Entire image  antialiasing=off  inType=Obsolete  imagePorts=One multidimensional signal  prodOutputMode=Binary point scaling  prodOutputWordLength=32  prodOutputFracLength=14  memoryMode=Specify word length  memoryWordLength=16  memoryFracLength=14  roundingMode=Floor  overflowMode=off
      settings: SourceProductName=Computer Vision System Toolbox
  Video Out : Outport
  wires:
  Bus Selector/2 -> Draw Shapes Red/2  "<red_bbox>"
  Bus Selector/1 -> Draw Shapes Green/2  "<green_bbox>"
  Draw Shapes Red/1 -> Video Out/1
  Draw Shapes Green/1 -> Draw Shapes Red/1
  Video In/1 -> Draw Shapes Green/1
  Blob Data/1 -> Bus Selector/1

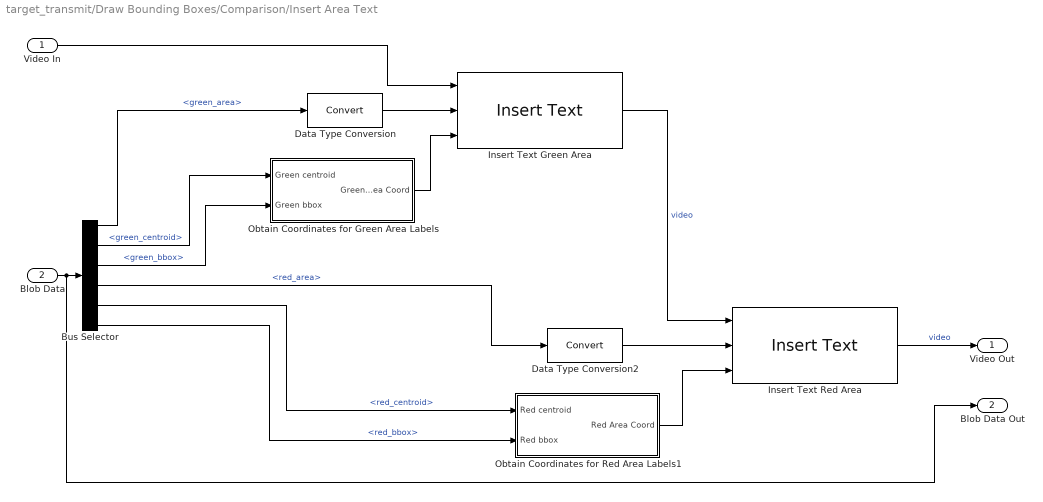
== system target_transmit/Draw Bounding Boxes/Comparison/Insert Area Text ==
  Video In : Inport
  Blob Data : Inport  Port=2
  Bus Selector : BusSelector  OutputSignals=green_area,green_centroid,green_bbox,red_area,red_centroid,red_bbox
  Data Type Conversion : DataTypeConversion
  Data Type Conversion2 : DataTypeConversion
  Insert Text Green Area : visiontextngfix/Insert Text  inputType=Obsolete  theText='Area: %d'  fontFace=LucidaSansRegular  dummyVar1=0  blockFontSize=12  antiAliased=on  getTextLocFrom=Input port  textLoc=[1 1]  getTextColorFrom=Specify via dialog  textColor=[0 255 0]  getTextIntensityFrom=Specify via dialog  textIntensity=0  getTextOpacityFrom=Specify via dialog  textOpacity=1.0  dummyVar2=0  dummyVar3=0  dummyVar4=0  imagePorts=One multidimensional signal  isInputTransposed=off
      settings: SourceProductName=Computer Vision System Toolbox  SourceProductBaseCode=VP
  Insert Text Red Area : visiontextngfix/Insert Text  inputType=Obsolete  theText='Area: %d'  fontFace=LucidaSansRegular  dummyVar1=0  blockFontSize=12  antiAliased=on  getTextLocFrom=Input port  textLoc=[1 1]  getTextColorFrom=Specify via dialog  textColor=[255 0 0]  getTextIntensityFrom=Specify via dialog  textIntensity=0  getTextOpacityFrom=Specify via dialog  textOpacity=1.0  dummyVar2=0  dummyVar3=0  dummyVar4=0  imagePorts=One multidimensional signal  isInputTransposed=off
      settings: SourceProductName=Computer Vision System Toolbox  SourceProductBaseCode=VP
  Obtain Coordinates for Green Area Labels : Subsystem
  Obtain Coordinates for Red Area Labels1 : Subsystem
  Video Out : Outport
  Blob Data Out : Outport  Port=2
  wires:
  Bus Selector/6 -> Obtain Coordinates for Red Area Labels1/2(Red bbox)  "<red_bbox>"
  Bus Selector/5 -> Obtain Coordinates for Red Area Labels1/1(Red centroid)  "<red_centroid>"
  Bus Selector/3 -> Obtain Coordinates for Green Area Labels/2(Green bbox)  "<green_bbox>"
  Bus Selector/2 -> Obtain Coordinates for Green Area Labels/1(Green centroid)  "<green_centroid>"
  Blob Data/1 -> Blob Data Out/1, Bus Selector/1
  Obtain Coordinates for Green Area Labels/1(Green Area Coord) -> Insert Text Green Area/3
  Data Type Conversion2/1 -> Insert Text Red Area/2
  Insert Text Green Area/1 -> Insert Text Red Area/1  "video"
  Obtain Coordinates for Red Area Labels1/1(Red Area Coord) -> Insert Text Red Area/3
  Data Type Conversion/1 -> Insert Text Green Area/2
  Bus Selector/1 -> Data Type Conversion/1  "<green_area>"
  Bus Selector/4 -> Data Type Conversion2/1  "<red_area>"
  Video In/1 -> Insert Text Green Area/1
  Insert Text Red Area/1 -> Video Out/1  "video"

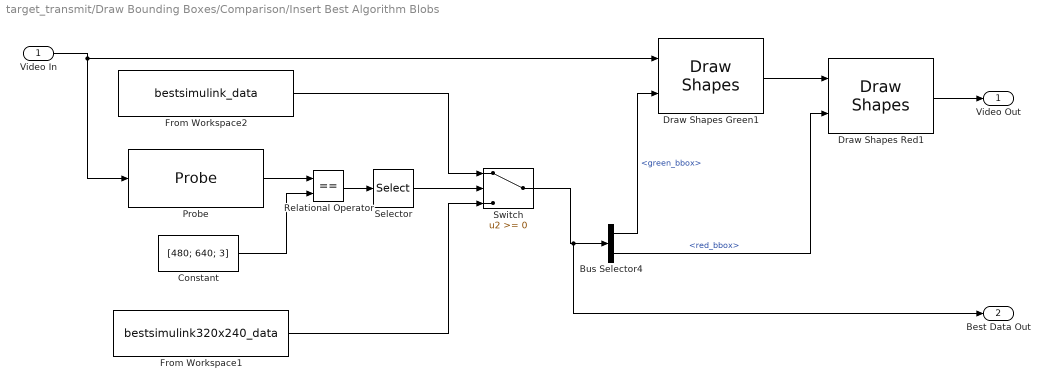
== system target_transmit/Draw Bounding Boxes/Comparison/Insert Best Algorithm Blobs ==
  Video In : Inport
  Bus Selector4 : BusSelector  OutputSignals=green_bbox,red_bbox
  Constant : Constant  Value=[480; 640; 3]
  Draw Shapes Green1 : visiontextngfix/Draw Shapes  shape=Rectangles  fill=on  lineWidth=1  fillClrSource=Specify via dialog  display=User-specified value  intensity=200  color=[0 255 0]  opacity=0.7  viewport=Entire image  antialiasing=off  inType=Obsolete  imagePorts=One multidimensional signal  prodOutputMode=Binary point scaling  prodOutputWordLength=32  prodOutputFracLength=14  memoryMode=Specify word length  memoryWordLength=16  memoryFracLength=14  roundingMode=Floor  overflowMode=off
      settings: SourceProductName=Computer Vision System Toolbox
  Draw Shapes Red1 : visiontextngfix/Draw Shapes  shape=Rectangles  fill=on  lineWidth=1  fillClrSource=Specify via dialog  display=User-specified value  intensity=200  color=[255 0 0]  opacity=0.7  viewport=Entire image  antialiasing=off  inType=Obsolete  imagePorts=One multidimensional signal  prodOutputMode=Binary point scaling  prodOutputWordLength=32  prodOutputFracLength=14  memoryMode=Specify word length  memoryWordLength=16  memoryFracLength=14  roundingMode=Floor  overflowMode=off
      settings: SourceProductName=Computer Vision System Toolbox
  From Workspace1 : FromWorkspace  VariableName=bestsimulink320x240_data  OutDataTypeStr=Bus: dataBusObject  SampleTime=0
  From Workspace2 : FromWorkspace  VariableName=bestsimulink_data  OutDataTypeStr=Bus: dataBusObject  SampleTime=0
  Probe : Probe  ProbeWidth=off  ProbeSampleTime=off  ProbeComplexSignal=off  ProbeSignalDimensions=on
  Relational Operator : RelationalOperator  Operator===  OutDataTypeStr=boolean  RndMeth=Nearest
  Selector : Selector  InputPortWidth=3  IndexOptions=Index vector (dialog)  Indices=1  OutputSizes=1
  Switch : Switch
  Video Out : Outport
  Best Data Out : Outport  Port=2
  wires:
  Draw Shapes Red1/1 -> Video Out/1
  Bus Selector4/2 -> Draw Shapes Red1/2  "<red_bbox>"
  Bus Selector4/1 -> Draw Shapes Green1/2  "<green_bbox>"
  Draw Shapes Green1/1 -> Draw Shapes Red1/1
  Video In/1 -> Probe/1, Draw Shapes Green1/1
  Probe/1 -> Relational Operator/1
  Constant/1 -> Relational Operator/2
  From Workspace1/1 -> Switch/3
  Relational Operator/1 -> Selector/1
  Selector/1 -> Switch/2
  From Workspace2/1 -> Switch/1
  Switch/1 -> Best Data Out/1, Bus Selector4/1

== system target_transmit/Draw Bounding Boxes/Comparison/Insert Closest Text ==
  Video In : Inport
  Blob Data : Inport  Port=2
  Bus Selector : BusSelector  OutputSignals=green_area,green_centroid,green_bbox,red_area,red_centroid,red_bbox
  Convert Bus to Double : Subsystem  Commented=on
  Find Closest Buoy : MATLAB Function  TreatAsAtomicUnit=on
  Insert Text Green Closest : visiontextngfix/Insert Text  inputType=Obsolete  theText='Closest Green Buoy'  getTextLocFrom=Input port  textLoc=[1 1]  getTextColorFrom=Specify via dialog  textColor=[0 255 0]  getTextIntensityFrom=Specify via dialog  textIntensity=0  getTextOpacityFrom=Specify via dialog  textOpacity=1.0  dummyVar2=0  dummyVar3=0  dummyVar4=0  imagePorts=One multidimensional signal  isInputTransposed=off  fontFace=LucidaSansRegular  dummyVar1=0  blockFontSize=12  antiAliased=on
      settings: SourceProductName=Computer Vision System Toolbox  SourceProductBaseCode=VP
  Insert Text Red Closest : visiontextngfix/Insert Text  inputType=Obsolete  theText='Closest Red Buoy'  getTextLocFrom=Input port  textLoc=[1 1]  getTextColorFrom=Specify via dialog  textColor=[255 0 0]  getTextIntensityFrom=Specify via dialog  textIntensity=0  getTextOpacityFrom=Specify via dialog  textOpacity=1.0  dummyVar2=0  dummyVar3=0  dummyVar4=0  imagePorts=One multidimensional signal  isInputTransposed=off  fontFace=LucidaSansRegular  dummyVar1=0  blockFontSize=12  antiAliased=on
      settings: SourceProductName=Computer Vision System Toolbox  SourceProductBaseCode=VP
  To Workspace : ToWorkspace  Commented=on  VariableName=data1  SaveFormat=Timeseries  SampleTime=-1
  Video Out : Outport
  wires:
  Convert Bus to Double/1(output) -> To Workspace/1
  Find Closest Buoy/3(data) -> Convert Bus to Double/1(input)
  Bus Selector/6 -> Find Closest Buoy/6(red_bbox)  "<red_bbox>"
  Bus Selector/1 -> Find Closest Buoy/1(green_area)  "<green_area>"
  Bus Selector/5 -> Find Closest Buoy/5(red_centroid)  "<red_centroid>"
  Bus Selector/2 -> Find Closest Buoy/2(green_centroid)  "<green_centroid>"
  Bus Selector/4 -> Find Closest Buoy/4(red_area)  "<red_area>"
  Bus Selector/3 -> Find Closest Buoy/3(green_bbox)  "<green_bbox>"
  Blob Data/1 -> Bus Selector/1
  Find Closest Buoy/2(rcoord) -> Insert Text Red Closest/2
  Find Closest Buoy/1(gcoord) -> Insert Text Green Closest/2
  Insert Text Red Closest/1 -> Video Out/1
  Video In/1 -> Insert Text Green Closest/1
  Insert Text Green Closest/1 -> Insert Text Red Closest/1

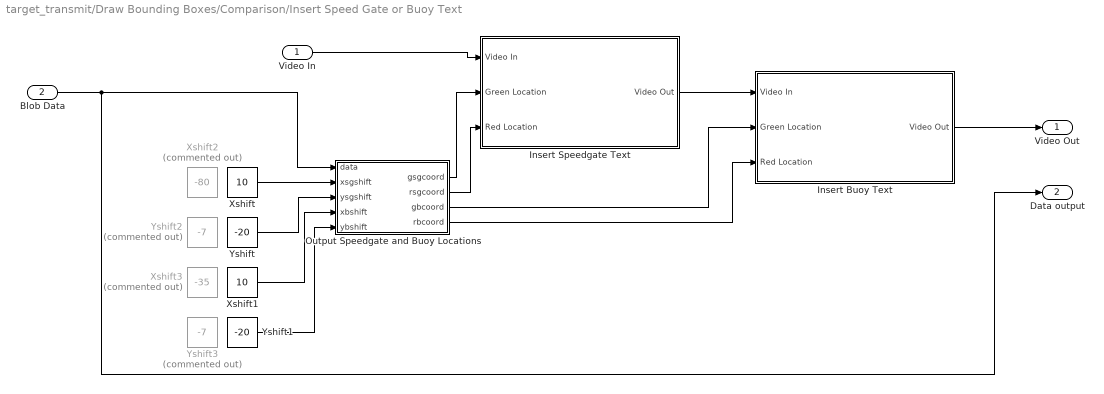
== system target_transmit/Draw Bounding Boxes/Comparison/Insert Speed Gate or Buoy Text ==
  Video In : Inport
  Blob Data : Inport  Port=2
  Insert Buoy Text : Subsystem
  Insert Speedgate Text : Subsystem
  Output Speedgate and Buoy Locations : MATLAB Function  TreatAsAtomicUnit=on
  Xshift : Constant  Value=10
  Xshift1 : Constant  Value=10
  Xshift2 : Constant  Commented=on  Value=-80
  Xshift3 : Constant  Commented=on  Value=-35
  Yshift : Constant  Value=-20
  Yshift1 : Constant  Value=-20
  Yshift2 : Constant  Commented=on  Value=-7
  Yshift3 : Constant  Commented=on  Value=-7
  Video Out : Outport
  Data output : Outport  Port=2
  wires:
  Blob Data/1 -> Output Speedgate and Buoy Locations/1(data), Data output/1
  Yshift1/1 -> Output Speedgate and Buoy Locations/5(ybshift)
  Xshift1/1 -> Output Speedgate and Buoy Locations/4(xbshift)
  Yshift/1 -> Output Speedgate and Buoy Locations/3(ysgshift)
  Xshift/1 -> Output Speedgate and Buoy Locations/2(xsgshift)
  Output Speedgate and Buoy Locations/4(rbcoord) -> Insert Buoy Text/3(Red Location)
  Output Speedgate and Buoy Locations/3(gbcoord) -> Insert Buoy Text/2(Green Location)
  Output Speedgate and Buoy Locations/2(rsgcoord) -> Insert Speedgate Text/3(Red Location)
  Output Speedgate and Buoy Locations/1(gsgcoord) -> Insert Speedgate Text/2(Green Location)
  Insert Buoy Text/1(Video Out) -> Video Out/1
  Insert Speedgate Text/1(Video Out) -> Insert Buoy Text/1(Video In)
  Video In/1 -> Insert Speedgate Text/1(Video In)

== system target_transmit/Draw Bounding Boxes/Comparison/Reflection Removal ==
  Blob Data In : Inport
  Bus Creator : BusCreator  Inputs=6
  Bus Selector2 : BusSelector  OutputSignals=green_area,green_centroid,green_bbox,red_area,red_centroid,red_bbox
  Green Reflection Removal : MATLAB Function  TreatAsAtomicUnit=on
  Red Reflection Removal : MATLAB Function  TreatAsAtomicUnit=on
  Blob Data Out : Outport
  wires:
  Red Reflection Removal/3(blob_bbox_out) -> Bus Creator/6  "red_bbox"
  Red Reflection Removal/1(blob_area_out) -> Bus Creator/4  "red_area"
  Red Reflection Removal/2(blob_centroid_out) -> Bus Creator/5  "red_centroid"
  Green Reflection Removal/3(blob_bbox_out) -> Bus Creator/3  "green_bbox"
  Green Reflection Removal/2(blob_centroid_out) -> Bus Creator/2  "green_centroid"
  Green Reflection Removal/1(blob_area_out) -> Bus Creator/1  "green_area"
  Bus Selector2/4 -> Red Reflection Removal/1(blob_area_in)  "<red_area>"
  Bus Selector2/6 -> Red Reflection Removal/3(blob_bbox_in)  "<red_bbox>"
  Bus Selector2/5 -> Red Reflection Removal/2(blob_centroid_in)  "<red_centroid>"
  Bus Selector2/3 -> Green Reflection Removal/3(blob_bbox_in)  "<green_bbox>"
  Bus Selector2/2 -> Green Reflection Removal/2(blob_centroid_in)  "<green_centroid>"
  Bus Selector2/1 -> Green Reflection Removal/1(blob_area_in)  "<green_area>"
  Blob Data In/1 -> Bus Selector2/1
  Bus Creator/1 -> Blob Data Out/1

== system target_transmit/Draw Bounding Boxes/No Comparison/Insert Area Text ==
  Video In : Inport
  Blob Data : Inport  Port=2
  Bus Selector : BusSelector  OutputSignals=green_area,green_centroid,green_bbox,red_area,red_centroid,red_bbox
  Data Type Conversion : DataTypeConversion
  Data Type Conversion2 : DataTypeConversion
  Insert Text Green Area : visiontextngfix/Insert Text  inputType=Obsolete  theText='Area: %d'  fontFace=LucidaSansRegular  dummyVar1=0  blockFontSize=12  antiAliased=on  getTextLocFrom=Input port  textLoc=[1 1]  getTextColorFrom=Specify via dialog  textColor=[0 255 0]  getTextIntensityFrom=Specify via dialog  textIntensity=0  getTextOpacityFrom=Specify via dialog  textOpacity=1.0  dummyVar2=0  dummyVar3=0  dummyVar4=0  imagePorts=One multidimensional signal  isInputTransposed=off
      settings: SourceProductName=Computer Vision System Toolbox  SourceProductBaseCode=VP
  Insert Text Red Area : visiontextngfix/Insert Text  inputType=Obsolete  theText='Area: %d'  fontFace=LucidaSansRegular  dummyVar1=0  blockFontSize=12  antiAliased=on  getTextLocFrom=Input port  textLoc=[1 1]  getTextColorFrom=Specify via dialog  textColor=[255 0 0]  getTextIntensityFrom=Specify via dialog  textIntensity=0  getTextOpacityFrom=Specify via dialog  textOpacity=1.0  dummyVar2=0  dummyVar3=0  dummyVar4=0  imagePorts=One multidimensional signal  isInputTransposed=off
      settings: SourceProductName=Computer Vision System Toolbox  SourceProductBaseCode=VP
  Obtain Coordinates for Green Area Labels : Subsystem
  Obtain Coordinates for Red Area Labels1 : Subsystem
  Video Out : Outport
  Blob Data Out : Outport  Port=2
  wires:
  Insert Text Red Area/1 -> Video Out/1  "video"
  Video In/1 -> Insert Text Green Area/1
  Bus Selector/4 -> Data Type Conversion2/1  "<red_area>"
  Bus Selector/1 -> Data Type Conversion/1  "<green_area>"
  Data Type Conversion/1 -> Insert Text Green Area/2
  Obtain Coordinates for Red Area Labels1/1(Red Area Coord) -> Insert Text Red Area/3
  Insert Text Green Area/1 -> Insert Text Red Area/1  "video"
  Data Type Conversion2/1 -> Insert Text Red Area/2
  Obtain Coordinates for Green Area Labels/1(Green Area Coord) -> Insert Text Green Area/3
  Blob Data/1 -> Blob Data Out/1, Bus Selector/1
  Bus Selector/2 -> Obtain Coordinates for Green Area Labels/1(Green centroid)  "<green_centroid>"
  Bus Selector/3 -> Obtain Coordinates for Green Area Labels/2(Green bbox)  "<green_bbox>"
  Bus Selector/5 -> Obtain Coordinates for Red Area Labels1/1(Red centroid)  "<red_centroid>"
  Bus Selector/6 -> Obtain Coordinates for Red Area Labels1/2(Red bbox)  "<red_bbox>"
